simulink model "RotationSimulation"  (R2016a)
settings: Solver=ode45  StartTime=0.0  StopTime=15  RelTol=1e-3
InitFcn:
  | RotSimu_initialization
StopFcn:
  | RotSimu_postprocessing
undefined symbols (not defined in the file or in its folder): initial_state, P
settings Model: Creator=eugensolowjow  LastModifiedBy=solowjow
settings DataIOCC: LimitDataPoints=on  SaveFormat=Array
settings DebuggingCC: SolverPrmCheckMsg=warning
settings HardwareCC: ProdBitPerPointer=32  ProdLargestAtomicFloat=None  ProdIntDivRoundTo=Undefined  ProdEndianess=Unspecified  ProdWordSize=32  ProdHWDeviceType=32-bit Generic
settings ModelReferenceCC: PropagateSignalLabelsOutOfModel=off
settings ConfigComp: CovModelRefEnable=Off  CovSFcnEnable=off

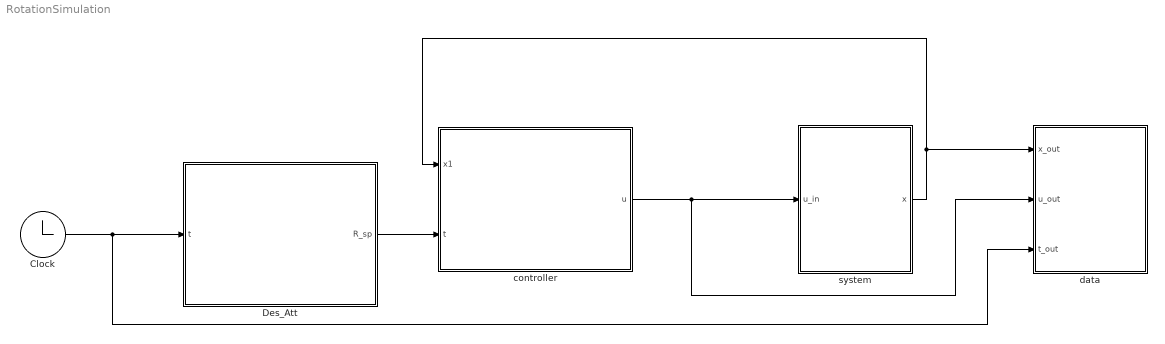
== system RotationSimulation ==
  Clock : Clock
  "Des_Att " : Subsystem
  controller : Subsystem
  data : Subsystem
  system : Subsystem
  wires:
  Clock/1 -> "Des_Att "/1(t), data/3(t_out)
  controller/1(u) -> system/1(u_in), data/2(u_out)
  system/1(x) -> data/1(x_out), controller/1(x1)
  "Des_Att "/1(R_sp) -> controller/2(t)

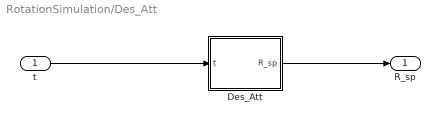
== system RotationSimulation/Des_Att  ==
  t : Inport
  Des_Att : MATLAB Function  TreatAsAtomicUnit=on
  R_sp : Outport
  wires:
  t/1 -> Des_Att/1(t)
  Des_Att/1(R_sp) -> R_sp/1

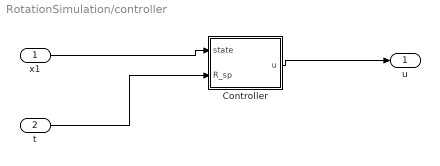
== system RotationSimulation/controller ==
  x1 : Inport
  t : Inport  Port=2
  Controller : MATLAB Function  TreatAsAtomicUnit=on
  u : Outport
  wires:
  t/1 -> Controller/2(R_sp)
  x1/1 -> Controller/1(state)
  Controller/1(u) -> u/1

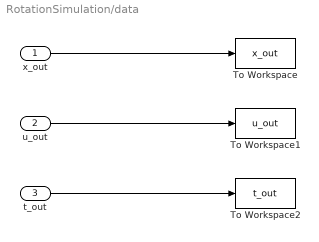
== system RotationSimulation/data ==
  x_out : Inport
  u_out : Inport  Port=2
  t_out : Inport  Port=3
  To Workspace : ToWorkspace  VariableName=x_out  SampleTime=-1
  To Workspace1 : ToWorkspace  VariableName=u_out  SampleTime=-1
  To Workspace2 : ToWorkspace  VariableName=t_out  SampleTime=-1
  wires:
  x_out/1 -> To Workspace/1
  u_out/1 -> To Workspace1/1
  t_out/1 -> To Workspace2/1

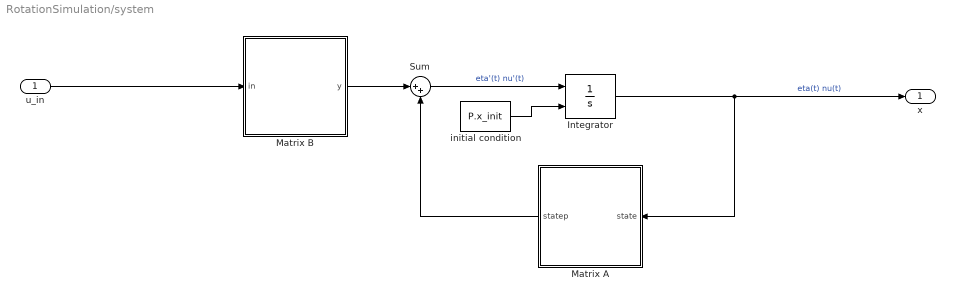
== system RotationSimulation/system ==
  u_in : Inport
  Integrator : Integrator  InitialConditionSource=external  InitialCondition=initial_state
  Matrix A : MATLAB Function  TreatAsAtomicUnit=on
  Matrix B : MATLAB Function  TreatAsAtomicUnit=on
  Sum : Sum  Inputs=|++
  initial condition : Constant  Value=P.x_init
  x : Outport
  wires:
  Matrix B/1(y) -> Sum/1
  Matrix A/1(statep) -> Sum/2
  Sum/1 -> Integrator/1  "eta'(t) nu'(t)"
  Integrator/1 -> x/1, Matrix A/1(state)  "eta(t) nu(t)"
  initial condition/1 -> Integrator/2
  u_in/1 -> Matrix B/1(in)

== matlab function RotationSimulation/Des_Att /Des_Att ==
  data: R_sp output; t input; P parameter
function R_sp = Des_Att(t,P)
%#codegen
phi = 0;
theta = 0;
psi = 0.3 * sin( 2*pi*t/3);

% Z-Y-X Euler angles to Rotation Matrx
R_sp = [cos(psi)*cos(theta),	(cos(psi)*sin(theta)*sin(phi) - sin(psi)*cos(phi)),	(sin(psi)*sin(phi)+cos(psi)*cos(phi)*sin(theta));
    sin(psi)*cos(theta),	(cos(phi)*cos(psi) + sin(phi)*sin(theta)*sin(psi)),	cos(phi)*sin(theta)*sin(psi)-cos(psi)*sin(phi); 
        -sin(theta),                        cos(theta)*sin(phi),                                cos(phi)*cos(theta)];

== matlab function RotationSimulation/controller/Controller ==
  data: state input; u output; R_sp input; P parameter
function u = Controller(state,R_sp,P)
%#codege
phi = state(1);
theta = state(2);
psi = state(3);
omega = [state(4); state(5); state(6)];

%inertia Tensor
J = diag([P.I_x, P.I_y, P.I_z]);

% Z-Y-X Euler angles to Rotation Matrx
R = [cos(psi)*cos(theta),	(cos(psi)*sin(theta)*sin(phi) - sin(psi)*cos(phi)),	(sin(psi)*sin(phi)+cos(psi)*cos(phi)*sin(theta));
    sin(psi)*cos(theta),	(cos(phi)*cos(psi) + sin(phi)*sin(theta)*sin(psi)),	cos(phi)*sin(theta)*sin(psi)-cos(psi)*sin(phi); 
        -sin(theta),                        cos(theta)*sin(phi),                                cos(phi)*cos(theta)];   
    

e_R = 0.5*(R_sp'*R - R'*R_sp);   %Compute attitude error

e_R_vec = [e_R(3,2); e_R(1,3); e_R(2,1)];   %vee-map the error to get a vector instead of matrix

torques = - P.Att_P_Gain * e_R_vec + cross(omega, J*omega);
u = torques;

== matlab function RotationSimulation/system/Matrix A ==
  data: state input; statep output; P parameter
function statep = fcn(state, P) %state = [eta, nu]' =[phi,theta,psi,p,q,r]'

phi = state(1);
theta = state(2);
psi = state(3);
p = state(4);
q = state(5);
r = state(6);

%rigid body mass matrix M_RB
M_RB = [ P.I_x,      -P.I_xy,    -P.I_xz;  
         -P.I_xy,    P.I_y,      P.I_yz;
         -P.I_xz,    -P.I_yz,    P.I_z];
   
   
   
% hydrodynamic added mass matrix M_A
%added mass matrix
M_A = [ P.K_pdot,   0,          0;
        0,          P.M_qdot,   0;
        0,          0,          P.N_rdot];
    

% damping matrix D
   
D =  [ P.K_p,	0,      0;
       0,      P.M_q,	0;
       0,      0,      P.N_r];
 
 
% rigid body coriolis matrix C_RB
C_RB = [    0,                          -P.I_yz*q-P.I_xz*p+P.I_z*r, P.I_yz*r+P.I_xy*p-P.I_y*q; 
            P.I_yz*q+P.I_xz*p-P.I_z*r,  0,                          -P.I_xz*r-P.I_xy*q+P.I_x*p;
            -P.I_yz*r-P.I_xy*p+P.I_y*q,  P.I_xz*r+P.I_xy*q-P.I_x*p,   0];
    

    
    %transformation matrix: angular velocities
J2 = [1,        sin(phi)*tan(theta),   cos(phi)*tan(theta); 
      0,        cos(phi),             -sin(phi); 
      0,        sin(phi)/cos(theta),   cos(phi)/cos(theta)];

%overall transformation matrix 
Jq = J2;   


    
%%%------------------------------------
    
%state-space model
A=[zeros(3,3),  Jq;
   zeros(3,3),  -inv(M_RB + M_A)*(C_RB + D)];

 
statep = A * state;

== matlab function RotationSimulation/system/Matrix B ==
  data: in input; y output; P parameter
function y = fcn(in, P)    %in = [p q r]

%rigid body mass matrix M_RB
M_RB = [ P.I_x,      -P.I_xy,    -P.I_xz;  
         -P.I_xy,    P.I_y,      P.I_yz;
         -P.I_xz,    -P.I_yz,    P.I_z];
   
   
% hydrodynamic added mass matrix M_A
%added mass matrix
M_A = [ P.K_pdot,   0,          0;
        0,          P.M_qdot,   0;
        0,          0,          P.N_rdot];
     
     
%matrix B for state-space model, size: 13x6
B=[zeros(3,3); inv(M_RB + M_A)];

y =  B*in;
